simulink model "t_d"  (R2019b)
settings: Solver=VariableStepAuto  StartTime=0.0  StopTime=10.0  RelTol=1e-3
model workspace (MAT data in the model file):
  K_b = 1
settings Model: Creator=jasper  LastModifiedBy=jasper

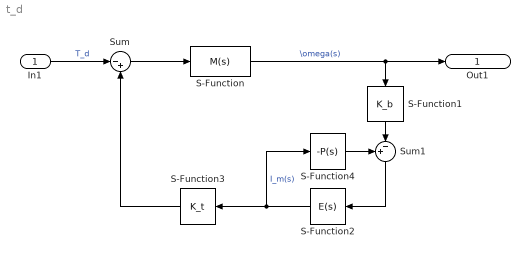
== system t_d ==
  In1 : Inport
  S-Function : S-Function  FunctionName=M(s)  SFunctionDeploymentMode=off  EnableBusSupport=off
  S-Function1 : S-Function  FunctionName=K_b  SFunctionDeploymentMode=off  EnableBusSupport=off
  S-Function2 : S-Function  FunctionName=E(s)  SFunctionDeploymentMode=off  EnableBusSupport=off
  S-Function3 : S-Function  FunctionName=K_t  SFunctionDeploymentMode=off  EnableBusSupport=off
  S-Function4 : S-Function  FunctionName=-P(s)  SFunctionDeploymentMode=off  EnableBusSupport=off
  Sum : Sum  Inputs=|-+
  Sum1 : Sum  Inputs=+-|
  Out1 : Outport
  wires:
  In1/1 -> Sum/1  "T_d"
  Sum/1 -> S-Function/1
  S-Function/1 -> S-Function1/1, Out1/1  "\\omega(s)"
  S-Function1/1 -> Sum1/2
  Sum1/1 -> S-Function2/1
  S-Function2/1 -> S-Function4/1, S-Function3/1  "I_m(s)"
  S-Function4/1 -> Sum1/1
  S-Function3/1 -> Sum/2
